simulink model "es2_sim"  (R2023b)
settings: Solver=VariableStepAuto  StartTime=0.0  StopTime=1000  RelTol=1e-3
values from neighbouring files (symbols this model uses):
  ueq = 0    [es2.m]
  x0 = [-0.1,0.1]'    [es2.m]
settings Model: Creator=stefa  LastModifiedBy=stefa

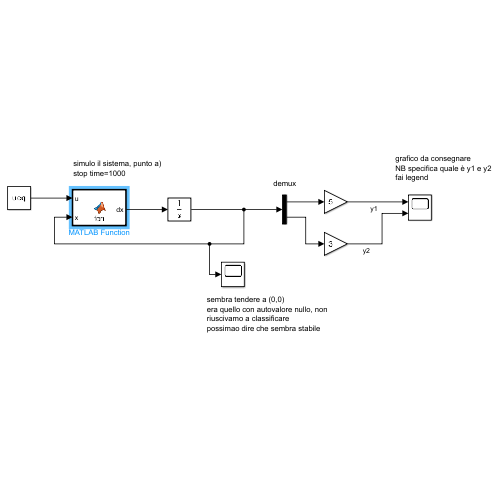
[thumbnail: Simulink's stored preview of the top-level diagram]
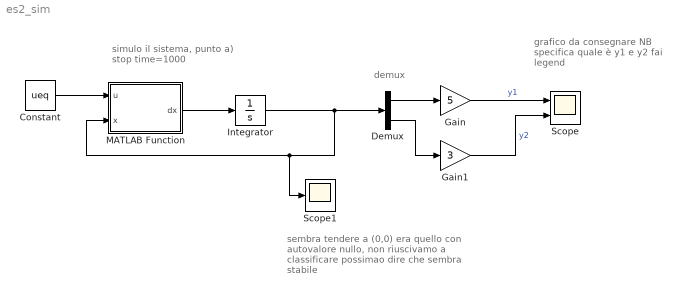
== system es2_sim ==
  note: grafico da consegnare
      | NB specifica quale è y1 e y2
      | fai legend
  note: sembra tendere a (0,0)
      | era quello con autovalore nullo, non riuscivamo a classificare
      | possimao dire che sembra stabile
  note: simulo il sistema, punto a)
      | stop time=1000
  note: demux
  Constant : Constant  Value=ueq
  Demux : Demux  Outputs=2
  Gain : Gain  Gain=5
  Gain1 : Gain  Gain=3
  Integrator : Integrator  InitialCondition=x0
  MATLAB Function : MATLAB Function  TreatAsAtomicUnit=on
  Scope : Scope  NumInputPorts=2
  Scope1 : Scope
  wires:
  Constant/1 -> MATLAB Function/1(u)
  MATLAB Function/1(dx) -> Integrator/1
  Integrator/1 -> Demux/1, Scope1/1, MATLAB Function/2(x)
  Demux/1 -> Gain/1
  Demux/2 -> Gain1/1
  Gain/1 -> Scope/1  "y1"
  Gain1/1 -> Scope/2  "y2"

== matlab function es2_sim/MATLAB Function ==
  data: u input; dx output; x input
function dx = fcn(u,x)
x1=x(1)
x2=x(2)
dx=[(x1^2+x1)*x2;-4*x2+x1-x2*u+3*u];
